simulink model "pfb_fir_real_test"  (Simulink 7.4)
settings: Solver=VariableStepDiscrete  StartTime=0.0  StopTime=500  RelTol=1e-3
libraries: xbsIndex_r4 x110
settings Model: Creator=User  LastModifiedBy=sgowda
settings OptimizationCC: InitFltsAndDblsToZero=on
settings DebuggingCC: SaveWithDisabledLinksMsg=none  SaveWithParameterizedLinksMsg=none

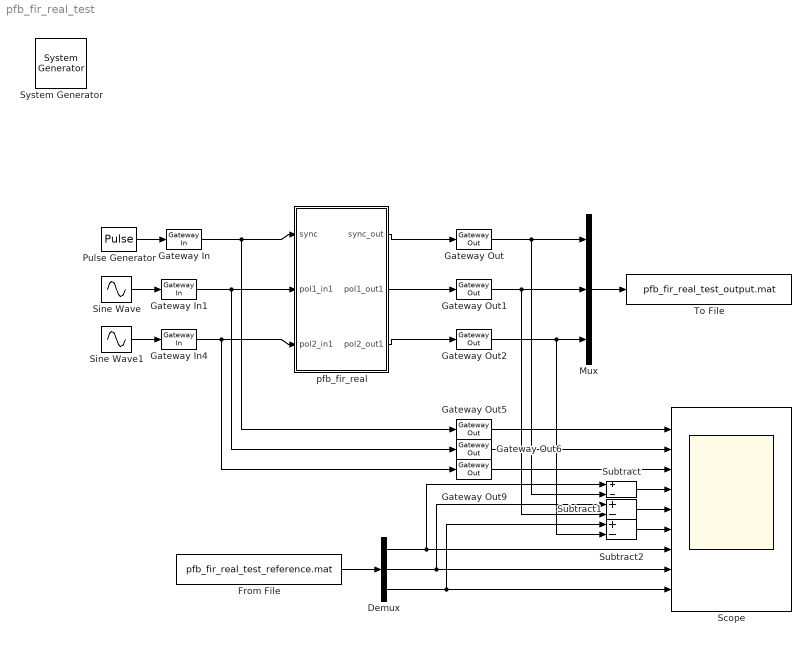
== system pfb_fir_real_test ==
  " System Generator" : xbsIndex_r4/ System Generator  Tag=genX  SystemSampleTime=-1  xilinxfamily=virtex4  part=xc4vsx35  speed=-10  package=ff668  synthesis_tool=XST  clock_wrapper=Clock Enables  directory=./netlist  testbench=off  simulink_period=1  sysclk_period=100  dcm_input_clock_period=100  incr_netlist=off  trim_vbits=Everywhere in SubSystem  dbl_ovrd=According to Block Masks  core_generation=According to Block Masks  run_coregen=off  deprecated_control=off  eval_field=0  block_type=sysgen
      settings: block_version=10.1.1
  Demux : Demux  Outputs=3
  From File : FromFile  FileName=pfb_fir_real_test_reference.mat  SampleTime=1
  Gateway In : xbsIndex_r4/Gateway In  arith_type=Boolean  n_bits=16  bin_pt=14  quantization="Round  (unbiased: +/- Inf)"  overflow=Saturate  period=1  dbl_ovrd=off  timing_constraint=None  locs_specified=off  LOCs={}  hdl_port=on  block_type=gatewayin
      settings: infoedit="Gateway in block.  Converts inputs of type Simulink integer, double and fixed point to  Xilinx fixed point type.<P><P>Hardware notes:  In hardware these blocks become top level input ports."  block_version=10.1.1
  Gateway In1 : xbsIndex_r4/Gateway In  arith_type="Signed  (2's comp)"  n_bits=10  bin_pt=9  quantization=Truncate  overflow=Wrap  period=1  dbl_ovrd=off  timing_constraint=None  locs_specified=off  LOCs={}  hdl_port=on  block_type=gatewayin
      settings: infoedit="Gateway in block.  Converts inputs of type Simulink integer, double and fixed point to  Xilinx fixed point type.<P><P>Hardware notes:  In hardware these blocks become top level input ports."  block_version=10.1.1
  Gateway In4 : xbsIndex_r4/Gateway In  arith_type="Signed  (2's comp)"  n_bits=10  bin_pt=9  quantization=Truncate  overflow=Wrap  period=1  dbl_ovrd=off  timing_constraint=None  locs_specified=off  LOCs={}  hdl_port=on  block_type=gatewayin
      settings: infoedit="Gateway in block.  Converts inputs of type Simulink integer, double and fixed point to  Xilinx fixed point type.<P><P>Hardware notes:  In hardware these blocks become top level input ports."  block_version=10.1.1
  Gateway Out{,1..2,5..6,9} (6 alike) : xbsIndex_r4/Gateway Out  hdl_port=on  timing_constraint=None  locs_specified=off  LOCs={}  block_type=gatewayout
      settings: infoedit="Gateway out block.  Converts Xilinx fixed point inputs into ouputs of type Simulink integer, double, or fixed point.<P><P>Hardware notes:  In hardware these blocks become top level output ports or are discarded, depending on how they are configured."  block_version=10.1.1
  Mux : Mux  Inputs=3
  Pulse Generator : DiscretePulseGenerator  Amplitude=1  Period=2^8  PulseWidth=1  PhaseDelay=13  SampleTime=1
  Scope : Scope  NumInputPorts=9
      settings: YMin=-5~-5~-5~-5~-5~-5~-5~-5~-5  YMax=5~5~5~5~5~5~5~5~5
  Sine Wave : Sin  SineType=Sample based  Amplitude=0.8  Bias=0  Frequency=1  Phase=0  Samples=16  SampleTime=1  Offset=7
  Sine Wave1 : Sin  SineType=Sample based  Amplitude=0.8  Bias=0  Frequency=1  Phase=0  Samples=8  SampleTime=1  Offset=7
  Subtract : Sum  Inputs=+-  OutDataType=fixdt(1, 16)  OutScaling=2^-10
  Subtract1 : Sum  Inputs=+-  OutDataType=fixdt(1, 16)  OutScaling=2^-10
  Subtract2 : Sum  Inputs=+-  OutDataType=fixdt(1, 16)  OutScaling=2^-10
  To File : ToFile  Filename=pfb_fir_real_test_output.mat  MatrixName=output
  pfb_fir_real : Subsystem  mask(pfb_fir_real){PFBSize=5, TotalTaps=5, WindowType=chebwin, n_inputs=0, MakeBiplex=1, BitWidthIn=10, BitWidthOut=22, CoeffBitWidth=10, CoeffDistMem=0, add_latency=2, mult_latency=3, bram_latency=1, conv_latency=2, quantization=Truncate, fwidth=0.80000000000000004440892098500626, specify_mult=off, mult_spec=[2                                      2], adder_folding=on, adder_tree_impl=Fabric}
      mask prompts: PFBSize "Size of PFB: (2^? pnts)"; TotalTaps "Total Number of Taps:"; WindowType "Windowing Function:"; n_inputs "Number of Simultaneous Inputs: (2^?)"; MakeBiplex "Make Biplex"; BitWidthIn "Input Bitwidth:"; BitWidthOut "Output Bitwidth:"; CoeffBitWidth "Coefficient Bitwidth:"; CoeffDistMem "Use Distributed Memory for Coeffs"; add_latency "Add Latency"; mult_latency "Mult Latency"; bram_latency "BRAM Latency"; conv_latency "Convert latency"; quantization "Quantization Behavior"; fwidth "Bin Width Scaling (normal=1)"; specify_mult "Specify multiplier use (behavioral if not specified)"; mult_spec "Multiplier specification (0=core, 1=embedded, 2=behavioural) (left=1st tap)"; adder_folding "Fold adders into DSPs"; adder_tree_impl "Adder implementation"
      mask help:
      | Fold adders into DSPs: Causes adders to be absorbed into DSP blocks (supported in Virtex5)
      | Adder implementation: Cores using Fabric or DSP48 or behavioral HDL
      mask init:
      | config.source = str2func('pfb_fir_init_xblock');
      | config.toplevel = gcb;
      | config.depend = {'pfb_fir_init_xblock.m', 'pfb_row_init_xblock.m', ...
      |     'adder_tree_init_xblock.m', 'macc_dsp48e_init_xblock.m', ...
      |     'pfb_coeff_gen_init_xblock.m', 'simd_add_dsp48e_init_xblock.m', ...
      |     'tap_multiply_fabric_init_xblock'};
      | if strcmp(specify_mult, 'on')
      |     mult_impl = 'DSP48e';
      | else
      |     mult_impl = 'Fabric';
      | end
      | xBlock(config, {PFBSize, TotalTaps, WindowType, ...
      |     n_inputs, MakeBiplex, BitWidthIn, BitWidthOut, ...
      |     CoeffBitWidth, CoeffDistMem, add_latency, mult_latency, ...
      |     bram_latency, conv_latency, quantization, fwidth, ...
      |     adder_tree_impl, mult_impl});
      settings: AttributesFormatString=taps=2, add_latency=1
      mask Help: eval('xlWeb(''http://casper.berkeley.edu/wiki/Pfb_fir_real'')')
      mask StyleString: edit,edit,popup(bartlett|barthannwin|blackman|blackmanharris|bohamwin|chebwin|flattopwin|gausswin|hamming|hann|kaiser|nuttallwin|parzenwin|rectwin|tukeywin|triang|userwindow),edit,edit,edit,edit,edit,edit,edit,edit,edit,edit,popup(Truncate|Round  (unbiased: +/- Inf)|Round  (unbiased: Even Values)),edit,checkbox,edit,checkbox,popup(Behavioral|Fabric|DSP48e)
      mask CallbackString:
      | |%num_taps = eval(get_param(gcb, 'TotalTaps'));
      | %old_vec = eval(get_param(gcb, 'mult_spec'));=-0l
      | 
      | %vec = 2.*ones(1,num_taps);
      | %old_size = length(old_vec);
      | 
      | %if(old_size <= num_taps),
      | %    new_size = old_size;
      | %else,
      | %    new_size = num_taps;
      | %end
      | 
      | %for n = 1:new_size, vec(n) = old_vec(n); end
      | %set_param(gcb, 'mult_spec', mat2str(vec));||||||||||||||%thisVariable = 'specify_mult';
      | %affectedVars = {'mult_spec'};
      | 
      | %thisBlock = gcb();
      | %thisVarState = get_param(thisBlock, thisVariable);
      | %maskNames = get_param(thisBlock, 'MaskNames');
      | %maskEnables = get_param(thisBlock, 'MaskEnables');
      | 
      | %for varName = affectedVars
      | %    varIndex = find(ismember(maskNames, varName));
      | %    maskEnables{varIndex} = thisVarState;
      | %end
      | 
      | %set_param(thisBlock, 'MaskEnables', maskEnables);|||
  wires:
  Pulse Generator/1 -> Gateway In/1
  Gateway In/1 -> Gateway Out5/1, pfb_fir_real/1(sync)
  Sine Wave/1 -> Gateway In1/1
  pfb_fir_real/1(sync_out) -> Gateway Out/1
  Sine Wave1/1 -> Gateway In4/1
  Gateway In1/1 -> Gateway Out6/1, pfb_fir_real/2(pol1_in1)
  Gateway In4/1 -> Gateway Out9/1, pfb_fir_real/3(pol2_in1)
  Gateway Out5/1 -> Scope/1
  Gateway Out6/1 -> Scope/2
  Gateway Out/1 -> Mux/1, Subtract/2
  Gateway Out1/1 -> Mux/2, Subtract1/2
  Gateway Out2/1 -> Mux/3, Subtract2/2
  Mux/1 -> To File/1
  pfb_fir_real/3(pol2_out1) -> Gateway Out2/1
  pfb_fir_real/2(pol1_out1) -> Gateway Out1/1
  Gateway Out9/1 -> Scope/3
  Subtract/1 -> Scope/4
  Subtract1/1 -> Scope/5
  Subtract2/1 -> Scope/6
  From File/1 -> Demux/1
  Demux/1 -> Scope/7, Subtract/1
  Demux/2 -> Scope/8, Subtract1/1
  Demux/3 -> Scope/9, Subtract2/1

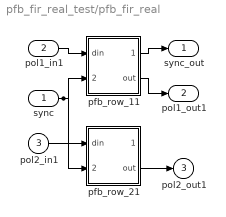
== system pfb_fir_real_test/pfb_fir_real ==
  sync : Inport
  pol1_in1 : Inport  Port=2
  pol2_in1 : Inport  Port=3
  pfb_row_11 : Subsystem
  pfb_row_21 : Subsystem
  sync_out : Outport
  pol1_out1 : Outport  Port=2
  pol2_out1 : Outport  Port=3
  wires:
  sync/1 -> pfb_row_21/2(sync), pfb_row_11/2(sync)
  pfb_row_21/2(out) -> pol2_out1/1
  pol2_in1/1 -> pfb_row_21/1(din)
  pfb_row_11/2(out) -> pol1_out1/1
  pfb_row_11/1(sync_out) -> sync_out/1
  pol1_in1/1 -> pfb_row_11/1(din)

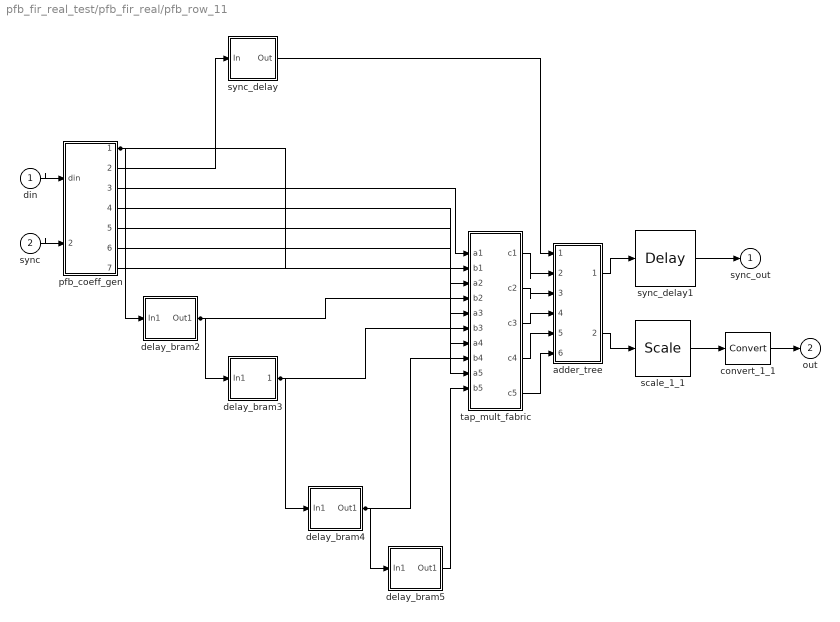
== system pfb_fir_real_test/pfb_fir_real/pfb_row_11 ==
  din : Inport
  sync : Inport  Port=2
  adder_tree : Subsystem
  convert_1_1 : xbsIndex_r4/Convert  arith_type="Signed  (2's comp)"  n_bits=22  bin_pt=21  quantization="Round  (unbiased: +/- Inf)"  overflow=Saturate  latency=1  dbl_ovrd=off  pipeline=on  block_type=convert
      settings: block_version=11.4
  delay_bram2 : Subsystem
  delay_bram3 : Subsystem
  delay_bram4 : Subsystem
  delay_bram5 : Subsystem
  pfb_coeff_gen : Subsystem
  scale_1_1 : xbsIndex_r4/Scale  scale_factor=-4  dbl_ovrd=off  block_type=scale
  sync_delay : Subsystem
  sync_delay1 : xbsIndex_r4/Delay  en=off  latency=2  dbl_ovrd=off  reg_retiming=off  block_type=delay
      settings: block_version=11.4
  tap_mult_fabric : Subsystem
  sync_out : Outport
  out : Outport  Port=2
  wires:
  pfb_coeff_gen/1(dout) -> tap_mult_fabric/2(b1), delay_bram2/1(In1)
  delay_bram2/1(Out1) -> tap_mult_fabric/4(b2), delay_bram3/1(In1)
  delay_bram3/1(Out1) -> tap_mult_fabric/6(b3), delay_bram4/1(In1)
  delay_bram4/1(Out1) -> tap_mult_fabric/8(b4), delay_bram5/1(In1)
  sync_delay/1(Out) -> adder_tree/1(sync)
  pfb_coeff_gen/2(sync_out) -> sync_delay/1(In)
  adder_tree/2(dout) -> scale_1_1/1
  adder_tree/1(sync_out) -> sync_delay1/1
  tap_mult_fabric/5(c5) -> adder_tree/6(din_5)
  tap_mult_fabric/4(c4) -> adder_tree/5(din_4)
  tap_mult_fabric/3(c3) -> adder_tree/4(din_3)
  tap_mult_fabric/2(c2) -> adder_tree/3(din_2)
  tap_mult_fabric/1(c1) -> adder_tree/2(din_1)
  delay_bram5/1(Out1) -> tap_mult_fabric/10(b5)
  pfb_coeff_gen/7(coeffs5) -> tap_mult_fabric/9(a5)
  pfb_coeff_gen/6(coeffs4) -> tap_mult_fabric/7(a4)
  pfb_coeff_gen/5(coeffs3) -> tap_mult_fabric/5(a3)
  pfb_coeff_gen/4(coeffs2) -> tap_mult_fabric/3(a2)
  pfb_coeff_gen/3(coeffs1) -> tap_mult_fabric/1(a1)
  sync_delay1/1 -> sync_out/1
  scale_1_1/1 -> convert_1_1/1
  convert_1_1/1 -> out/1
  sync/1 -> pfb_coeff_gen/2(sync)
  din/1 -> pfb_coeff_gen/1(din)

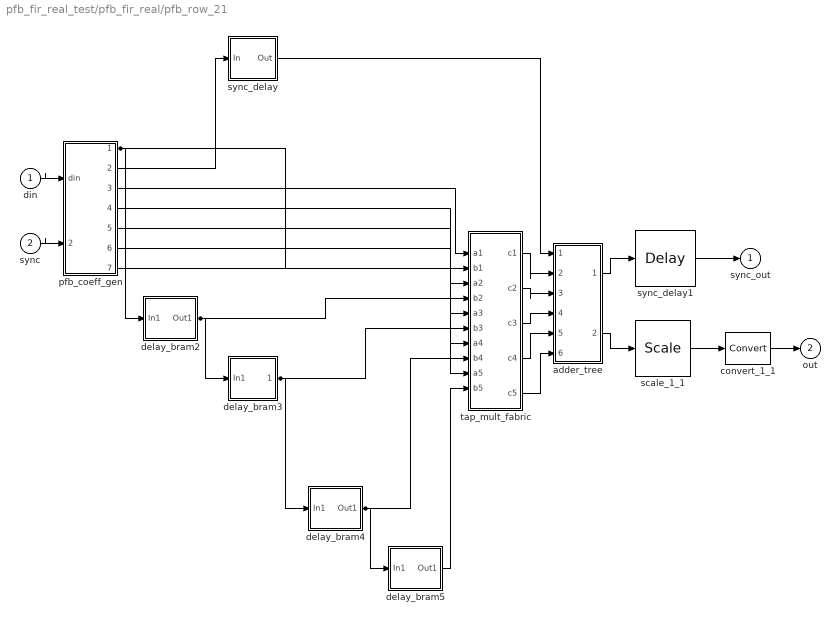
== system pfb_fir_real_test/pfb_fir_real/pfb_row_21 ==
  din : Inport
  sync : Inport  Port=2
  adder_tree : Subsystem
  convert_1_1 : xbsIndex_r4/Convert  arith_type="Signed  (2's comp)"  n_bits=22  bin_pt=21  quantization="Round  (unbiased: +/- Inf)"  overflow=Saturate  latency=1  dbl_ovrd=off  pipeline=on  block_type=convert
      settings: block_version=11.4
  delay_bram2 : Subsystem
  delay_bram3 : Subsystem
  delay_bram4 : Subsystem
  delay_bram5 : Subsystem
  pfb_coeff_gen : Subsystem
  scale_1_1 : xbsIndex_r4/Scale  scale_factor=-4  dbl_ovrd=off  block_type=scale
  sync_delay : Subsystem
  sync_delay1 : xbsIndex_r4/Delay  en=off  latency=2  dbl_ovrd=off  reg_retiming=off  block_type=delay
      settings: block_version=11.4
  tap_mult_fabric : Subsystem
  sync_out : Outport
  out : Outport  Port=2
  wires:
  pfb_coeff_gen/1(dout) -> tap_mult_fabric/2(b1), delay_bram2/1(In1)
  delay_bram2/1(Out1) -> tap_mult_fabric/4(b2), delay_bram3/1(In1)
  delay_bram3/1(Out1) -> tap_mult_fabric/6(b3), delay_bram4/1(In1)
  delay_bram4/1(Out1) -> tap_mult_fabric/8(b4), delay_bram5/1(In1)
  sync_delay/1(Out) -> adder_tree/1(sync)
  pfb_coeff_gen/2(sync_out) -> sync_delay/1(In)
  adder_tree/2(dout) -> scale_1_1/1
  adder_tree/1(sync_out) -> sync_delay1/1
  tap_mult_fabric/5(c5) -> adder_tree/6(din_5)
  tap_mult_fabric/4(c4) -> adder_tree/5(din_4)
  tap_mult_fabric/3(c3) -> adder_tree/4(din_3)
  tap_mult_fabric/2(c2) -> adder_tree/3(din_2)
  tap_mult_fabric/1(c1) -> adder_tree/2(din_1)
  delay_bram5/1(Out1) -> tap_mult_fabric/10(b5)
  pfb_coeff_gen/7(coeffs5) -> tap_mult_fabric/9(a5)
  pfb_coeff_gen/6(coeffs4) -> tap_mult_fabric/7(a4)
  pfb_coeff_gen/5(coeffs3) -> tap_mult_fabric/5(a3)
  pfb_coeff_gen/4(coeffs2) -> tap_mult_fabric/3(a2)
  pfb_coeff_gen/3(coeffs1) -> tap_mult_fabric/1(a1)
  sync_delay1/1 -> sync_out/1
  scale_1_1/1 -> convert_1_1/1
  convert_1_1/1 -> out/1
  sync/1 -> pfb_coeff_gen/2(sync)
  din/1 -> pfb_coeff_gen/1(din)

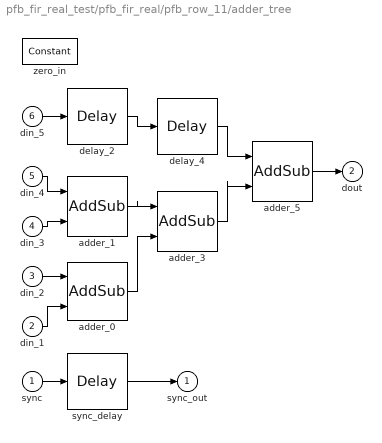
== system pfb_fir_real_test/pfb_fir_real/pfb_row_11/adder_tree ==
  sync : Inport
  din_1 : Inport  Port=2
  din_2 : Inport  Port=3
  din_3 : Inport  Port=4
  din_4 : Inport  Port=5
  din_5 : Inport  Port=6
  adder_{0..1,3,5} (4 alike) : xbsIndex_r4/AddSub  mode=Addition  use_carryin=off  use_carryout=off  en=off  latency=2  precision=Full  arith_type=Unsigned  n_bits=16  bin_pt=14  quantization=Truncate  overflow=Wrap  dbl_ovrd=off  use_behavioral_HDL=off  hw_selection=Fabric  pipelined=off  block_type=addsub
  delay_2 : xbsIndex_r4/Delay  en=off  latency=2  dbl_ovrd=off  reg_retiming=off  block_type=delay
      settings: block_version=11.4
  delay_4 : xbsIndex_r4/Delay  en=off  latency=2  dbl_ovrd=off  reg_retiming=off  block_type=delay
      settings: block_version=11.4
  sync_delay : xbsIndex_r4/Delay  en=off  latency=6  dbl_ovrd=off  reg_retiming=off  block_type=delay
      settings: block_version=11.4
  zero_in : xbsIndex_r4/Constant  arith_type=Unsigned  const=0  n_bits=18  bin_pt=17  explicit_period=off  period=1  equ=P=C  opselect=C  inp2=PCIN>>17  opr=+  inp1=P  carry=CIN  dbl_ovrd=off  block_type=constant
      settings: block_version=11.4
  sync_out : Outport
  dout : Outport  Port=2
  wires:
  adder_5/1 -> dout/1
  adder_3/1 -> adder_5/2
  delay_4/1 -> adder_5/1
  delay_2/1 -> delay_4/1
  adder_0/1 -> adder_3/2
  adder_1/1 -> adder_3/1
  din_5/1 -> delay_2/1
  din_3/1 -> adder_1/2
  din_4/1 -> adder_1/1
  din_1/1 -> adder_0/2
  din_2/1 -> adder_0/1
  sync_delay/1 -> sync_out/1
  sync/1 -> sync_delay/1

== system pfb_fir_real_test/pfb_fir_real/pfb_row_11/delay_bram2 ==
  In1 : Inport
  Constant2 : xbsIndex_r4/Constant  arith_type=Boolean  const=1  n_bits=1  bin_pt=0  explicit_period=on  period=1  equ=P=C  opselect=C  inp2=PCIN>>17  opr=+  inp1=P  carry=CIN  dbl_ovrd=off  block_type=constant
      settings: block_version=11.4
  Counter : xbsIndex_r4/Counter  cnt_type=Count Limited  cnt_to=30  operation=Up  start_count=0  cnt_by_val=1  arith_type=Unsigned  n_bits=5  bin_pt=0  load_pin=off  rst=off  en=off  explicit_period=on  period=1  dbl_ovrd=off  use_behavioral_HDL=off  implementation=DSP48  use_rpm=on  block_type=counter
      settings: block_version=11.4
  Single Port RAM : xbsIndex_r4/Single Port RAM  depth=32  initVector=0  distributed_mem=Block RAM  write_mode=Read Before Write  rst=off  init_reg=0  en=off  latency=1  dbl_ovrd=off  optimize=Area  use_rpm=off  block_type=spram
  Out1 : Outport
  wires:
  Single Port RAM/1 -> Out1/1
  Constant2/1 -> Single Port RAM/3
  In1/1 -> Single Port RAM/2
  Counter/1 -> Single Port RAM/1

== system pfb_fir_real_test/pfb_fir_real/pfb_row_11/delay_bram3 ==
  In1 : Inport
  Constant2 : xbsIndex_r4/Constant  arith_type=Boolean  const=1  n_bits=1  bin_pt=0  explicit_period=on  period=1  equ=P=C  opselect=C  inp2=PCIN>>17  opr=+  inp1=P  carry=CIN  dbl_ovrd=off  block_type=constant
      settings: block_version=11.4
  Counter : xbsIndex_r4/Counter  cnt_type=Count Limited  cnt_to=30  operation=Up  start_count=0  cnt_by_val=1  arith_type=Unsigned  n_bits=5  bin_pt=0  load_pin=off  rst=off  en=off  explicit_period=on  period=1  dbl_ovrd=off  use_behavioral_HDL=off  implementation=DSP48  use_rpm=on  block_type=counter
      settings: block_version=11.4
  Single Port RAM : xbsIndex_r4/Single Port RAM  depth=32  initVector=0  distributed_mem=Block RAM  write_mode=Read Before Write  rst=off  init_reg=0  en=off  latency=1  dbl_ovrd=off  optimize=Area  use_rpm=off  block_type=spram
  Out1 : Outport
  wires:
  Single Port RAM/1 -> Out1/1
  Constant2/1 -> Single Port RAM/3
  In1/1 -> Single Port RAM/2
  Counter/1 -> Single Port RAM/1

== system pfb_fir_real_test/pfb_fir_real/pfb_row_11/delay_bram4 ==
  In1 : Inport
  Constant2 : xbsIndex_r4/Constant  arith_type=Boolean  const=1  n_bits=1  bin_pt=0  explicit_period=on  period=1  equ=P=C  opselect=C  inp2=PCIN>>17  opr=+  inp1=P  carry=CIN  dbl_ovrd=off  block_type=constant
      settings: block_version=11.4
  Counter : xbsIndex_r4/Counter  cnt_type=Count Limited  cnt_to=30  operation=Up  start_count=0  cnt_by_val=1  arith_type=Unsigned  n_bits=5  bin_pt=0  load_pin=off  rst=off  en=off  explicit_period=on  period=1  dbl_ovrd=off  use_behavioral_HDL=off  implementation=DSP48  use_rpm=on  block_type=counter
      settings: block_version=11.4
  Single Port RAM : xbsIndex_r4/Single Port RAM  depth=32  initVector=0  distributed_mem=Block RAM  write_mode=Read Before Write  rst=off  init_reg=0  en=off  latency=1  dbl_ovrd=off  optimize=Area  use_rpm=off  block_type=spram
  Out1 : Outport
  wires:
  Single Port RAM/1 -> Out1/1
  Constant2/1 -> Single Port RAM/3
  In1/1 -> Single Port RAM/2
  Counter/1 -> Single Port RAM/1

== system pfb_fir_real_test/pfb_fir_real/pfb_row_11/delay_bram5 ==
  In1 : Inport
  Constant2 : xbsIndex_r4/Constant  arith_type=Boolean  const=1  n_bits=1  bin_pt=0  explicit_period=on  period=1  equ=P=C  opselect=C  inp2=PCIN>>17  opr=+  inp1=P  carry=CIN  dbl_ovrd=off  block_type=constant
      settings: block_version=11.4
  Counter : xbsIndex_r4/Counter  cnt_type=Count Limited  cnt_to=30  operation=Up  start_count=0  cnt_by_val=1  arith_type=Unsigned  n_bits=5  bin_pt=0  load_pin=off  rst=off  en=off  explicit_period=on  period=1  dbl_ovrd=off  use_behavioral_HDL=off  implementation=DSP48  use_rpm=on  block_type=counter
      settings: block_version=11.4
  Single Port RAM : xbsIndex_r4/Single Port RAM  depth=32  initVector=0  distributed_mem=Block RAM  write_mode=Read Before Write  rst=off  init_reg=0  en=off  latency=1  dbl_ovrd=off  optimize=Area  use_rpm=off  block_type=spram
  Out1 : Outport
  wires:
  Single Port RAM/1 -> Out1/1
  Constant2/1 -> Single Port RAM/3
  In1/1 -> Single Port RAM/2
  Counter/1 -> Single Port RAM/1

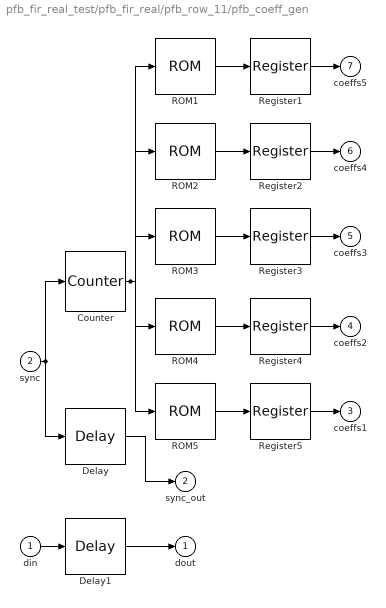
== system pfb_fir_real_test/pfb_fir_real/pfb_row_11/pfb_coeff_gen ==
  din : Inport
  sync : Inport  Port=2
  Counter : xbsIndex_r4/Counter  cnt_type=Free Running  cnt_to=Inf  operation=Up  start_count=0  cnt_by_val=1  arith_type=Unsigned  n_bits=5  bin_pt=0  load_pin=off  rst=on  en=off  explicit_period=on  period=1  dbl_ovrd=off  use_behavioral_HDL=off  implementation=Fabric  use_rpm=on  block_type=counter
      settings: block_version=11.4
  Delay : xbsIndex_r4/Delay  en=off  latency=2  dbl_ovrd=off  reg_retiming=off  block_type=delay
      settings: block_version=11.4
  Delay1 : xbsIndex_r4/Delay  en=off  latency=3  dbl_ovrd=off  reg_retiming=off  block_type=delay
      settings: block_version=11.4
  ROM1 : xbsIndex_r4/ROM  depth=32  initVector=[-1.83537948689192e-20 -5.5570212494937e-06 -1.63600419269467e-05 -3.47242296265235e-05 -6.35238166447315e-05 -0.000106241976471681 -0.000167008217876277 -0.000250618800937326 -0.000362535388329735 -0.000508856971932249 -0.000696260082747423 -0.000931902422689507 -0.00122328536860849 -0.00157807130674446 -0.00200385246963349 -0.002507868871658 -0.00309667407189773 -0.00377574882462827 -0.00454906419223727 -0.00541859736832988 -0.00638380525859058 -0.00744106275440964 -0.00858307456340268 -0.00979827137977639 -0.011070203029117 -0.0123769429460894 -0.0136905198771712 -0.0149763939810333 -0.0161929954652235 -0.017291344491685 -0.0182147712532231 -0.0188987548237974]  distributed_mem=Block RAM  rst=off  init_reg=0  en=off  latency=2  arith_type="Signed  (2's comp)"  n_bits=10  bin_pt=9  dbl_ovrd=off  optimize=Area  use_rpm=on  block_type=sprom
      settings: block_version=11.4
  ROM2 : xbsIndex_r4/ROM  depth=32  initVector=[-0.0192708985824556 -0.0192510586801436 -0.0187516401496287 -0.0176780728545899 -0.0159294765527955 -0.013399520943983 -0.00997748273503472 -0.00554949754803241 9.58776090258162e-18 0.00678665941101795 0.0149244367666534 0.024523677457147 0.0356890847292955 0.0485176039711326 0.0630962566317489 0.0794999611480237 0.0977893811012691 0.118008842950763 0.140184366995717 0.164321855626379 0.190405482381545 0.21839632379788 0.248231273503403 0.279822274484999 0.313055900984824 0.34779331611502 0.383870625110952 0.421099637279897 0.459269042275782 0.498145998490477 0.537478123262804 0.576995866443847]  distributed_mem=Block RAM  rst=off  init_reg=0  en=off  latency=2  arith_type="Signed  (2's comp)"  n_bits=10  bin_pt=9  dbl_ovrd=off  optimize=Area  use_rpm=on  block_type=sprom
      settings: block_version=11.4
  ROM3 : xbsIndex_r4/ROM  depth=32  initVector=[0.616415240804449 0.655440875013837 0.693769347641133 0.731092754011235 0.767102451949175 0.80149292762253 0.83396571896988 0.864233331691149 0.892023081552472 0.917080796874454 0.939174316547831 0.958096721742031 0.973669243595624 0.98574379452744 0.99420507727783 0.998972233248538 1 0.997279356709406 0.990837645797992 0.980738168597035 0.967079262627824 0.949992877609162 0.929642676468857 0.906221696224427 0.879949611428438 0.851069649779872 0.819845215341666 0.786556279459168 0.751495602856677 0.714964854442019 0.67727069304653 0.638720877676221]  distributed_mem=Block RAM  rst=off  init_reg=0  en=off  latency=2  arith_type="Signed  (2's comp)"  n_bits=10  bin_pt=9  dbl_ovrd=off  optimize=Area  use_rpm=on  block_type=sprom
      settings: block_version=11.4
  ROM4 : xbsIndex_r4/ROM  depth=32  initVector=[0.599620469886999 0.560268188690169 0.520952974039709 0.481950809570252 0.443521848986383 0.40590788350912 0.369330180237019 0.333987713358341 0.300055802042386 0.267685160726547 0.237001359579851 0.208104685332775 0.181070385572542 0.155949273151139 0.132768661658431 0.111533598070868 0.0922283547694533 0.0748181401760309 0.0592509853065098 0.0454597625806334 0.0333642932339546 0.0228735006003976 0.0138875683049731 0.00630006494050392 8.87861210313256e-18 -0.00512622041298097 -0.00919296538822508 -0.0123137013214723 -0.0145994824432491 -0.0161576231160187 -0.0170905605431562 -0.017494911978617]  distributed_mem=Block RAM  rst=off  init_reg=0  en=off  latency=2  arith_type="Signed  (2's comp)"  n_bits=10  bin_pt=9  dbl_ovrd=off  optimize=Area  use_rpm=on  block_type=sprom
      settings: block_version=11.4
  ROM5 : xbsIndex_r4/ROM  depth=32  initVector=[-0.017460726222102 -0.0170709252152087 -0.0164009279898009 -0.0155184461159748 -0.0144834371934731 -0.013348200851566 -0.0121576001774965 -0.0109493904773777 -0.00975463676747319 -0.00859820136776993 -0.00749928338318453 -0.00647199266182947 -0.00552594195933946 -0.00466684245382657 -0.00389708938574173 -0.00321632637849668 -0.00262197886823068 -0.00210974897665909 -0.00167406604597449 -0.00130848887129482 -0.00100605737264354 -0.000759593010482301 -0.000561948639457462 -0.000406209694920779 -0.000285849604064716 -0.000194843103417715 -0.000127741728803638 -7.97161304010817e-05 -4.65700670323589e-05 -2.47309672256418e-05 -1.12218300973319e-05 -5.95375857785367e-06]  distributed_mem=Block RAM  rst=off  init_reg=0  en=off  latency=2  arith_type="Signed  (2's comp)"  n_bits=10  bin_pt=9  dbl_ovrd=off  optimize=Area  use_rpm=on  block_type=sprom
      settings: block_version=11.4
  Register{1..5} (5 alike) : xbsIndex_r4/Register  init=0  rst=off  en=off  dbl_ovrd=off  block_type=register
      settings: block_version=11.4
  dout : Outport
  sync_out : Outport  Port=2
  coeffs1 : Outport  Port=3
  coeffs2 : Outport  Port=4
  coeffs3 : Outport  Port=5
  coeffs4 : Outport  Port=6
  coeffs5 : Outport  Port=7
  wires:
  sync/1 -> Delay/1, Counter/1
  Counter/1 -> ROM1/1, ROM2/1, ROM3/1, ROM4/1, ROM5/1
  Register1/1 -> coeffs5/1
  ROM1/1 -> Register1/1
  Register2/1 -> coeffs4/1
  ROM2/1 -> Register2/1
  Register3/1 -> coeffs3/1
  ROM3/1 -> Register3/1
  Register4/1 -> coeffs2/1
  ROM4/1 -> Register4/1
  Register5/1 -> coeffs1/1
  ROM5/1 -> Register5/1
  Delay1/1 -> dout/1
  din/1 -> Delay1/1
  Delay/1 -> sync_out/1

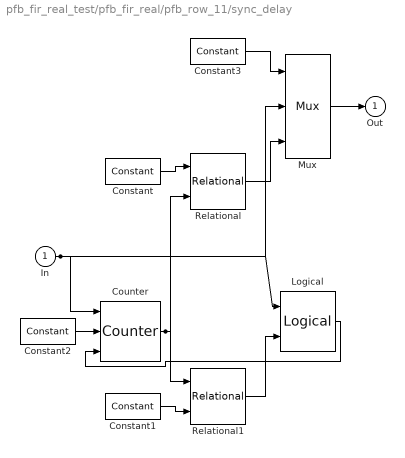
== system pfb_fir_real_test/pfb_fir_real/pfb_row_11/sync_delay ==
  In : Inport
  Constant : xbsIndex_r4/Constant  arith_type=Unsigned  const=1  n_bits=8  bin_pt=0  explicit_period=on  period=1  equ=P=C  opselect=C  inp2=PCIN>>17  opr=+  inp1=P  carry=CIN  dbl_ovrd=off  block_type=constant
      settings: block_version=11.4
  Constant1 : xbsIndex_r4/Constant  arith_type=Unsigned  const=0  n_bits=8  bin_pt=0  explicit_period=on  period=1  equ=P=C  opselect=C  inp2=PCIN>>17  opr=+  inp1=P  carry=CIN  dbl_ovrd=off  block_type=constant
      settings: block_version=11.4
  Constant2 : xbsIndex_r4/Constant  arith_type=Unsigned  const=131  n_bits=8  bin_pt=0  explicit_period=on  period=1  equ=P=C  opselect=C  inp2=PCIN>>17  opr=+  inp1=P  carry=CIN  dbl_ovrd=off  block_type=constant
      settings: block_version=11.4
  Constant3 : xbsIndex_r4/Constant  arith_type=Unsigned  const=1  n_bits=1  bin_pt=0  explicit_period=on  period=1  equ=P=C  opselect=C  inp2=PCIN>>17  opr=+  inp1=P  carry=CIN  dbl_ovrd=off  block_type=constant
      settings: block_version=11.4
  Counter : xbsIndex_r4/Counter  cnt_type=Free Running  cnt_to=Inf  operation=Down  start_count=0  cnt_by_val=1  arith_type=Unsigned  n_bits=8  bin_pt=0  load_pin=on  rst=off  en=on  explicit_period=on  period=1  dbl_ovrd=off  use_behavioral_HDL=off  implementation=Fabric  use_rpm=on  block_type=counter
      settings: block_version=11.4
  Logical : xbsIndex_r4/Logical  logical_function=OR  inputs=2  en=off  latency=0  precision=Full  arith_type=Unsigned  n_bits=16  bin_pt=0  align_bp=on  dbl_ovrd=off  block_type=logical
      settings: block_version=11.4
  Mux : xbsIndex_r4/Mux  inputs=2  en=off  latency=0  precision=Full  arith_type="Signed  (2's comp)"  n_bits=8  bin_pt=2  quantization=Truncate  overflow=Wrap  dbl_ovrd=off  block_type=mux
      settings: block_version=11.4
  Relational : xbsIndex_r4/Relational  mode=a=b  en=off  latency=0  dbl_ovrd=off  block_type=relational
  Relational1 : xbsIndex_r4/Relational  mode=a!=b  en=off  latency=0  dbl_ovrd=off  block_type=relational
  Out : Outport
  wires:
  In/1 -> Mux/2, Logical/1, Counter/1
  Counter/1 -> Relational1/1, Relational/2
  Relational1/1 -> Logical/2
  Constant1/1 -> Relational1/2
  Relational/1 -> Mux/3
  Constant/1 -> Relational/1
  Mux/1 -> Out/1
  Constant3/1 -> Mux/1
  Logical/1 -> Counter/3
  Constant2/1 -> Counter/2

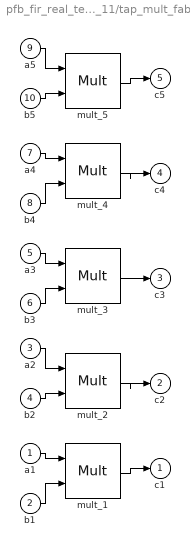
== system pfb_fir_real_test/pfb_fir_real/pfb_row_11/tap_mult_fabric ==
  a1 : Inport
  b1 : Inport  Port=2
  a2 : Inport  Port=3
  b2 : Inport  Port=4
  a3 : Inport  Port=5
  b3 : Inport  Port=6
  a4 : Inport  Port=7
  b4 : Inport  Port=8
  a5 : Inport  Port=9
  b5 : Inport  Port=10
  mult_{1..5} (5 alike) : xbsIndex_r4/Mult  precision=Full  arith_type="Signed  (2's comp)"  n_bits=16  bin_pt=14  quantization=Truncate  overflow=Wrap  en=off  latency=3  dbl_ovrd=off  use_behavioral_HDL=off  opt=Speed  use_embedded=on  optimum_pipeline=off  pipeline=on  use_rpm=on  placement_style=Triangular  block_type=mult
      settings: block_version=11.4
  c1 : Outport
  c2 : Outport  Port=2
  c3 : Outport  Port=3
  c4 : Outport  Port=4
  c5 : Outport  Port=5
  wires:
  mult_5/1 -> c5/1
  b5/1 -> mult_5/2
  a5/1 -> mult_5/1
  mult_4/1 -> c4/1
  b4/1 -> mult_4/2
  a4/1 -> mult_4/1
  mult_3/1 -> c3/1
  b3/1 -> mult_3/2
  a3/1 -> mult_3/1
  mult_2/1 -> c2/1
  b2/1 -> mult_2/2
  a2/1 -> mult_2/1
  mult_1/1 -> c1/1
  b1/1 -> mult_1/2
  a1/1 -> mult_1/1

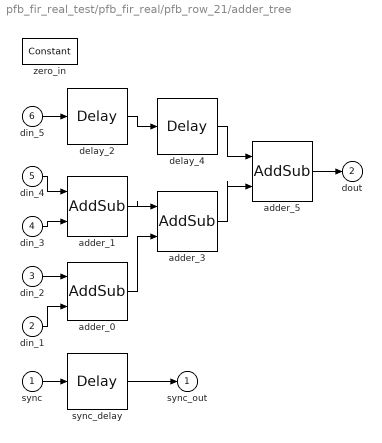
== system pfb_fir_real_test/pfb_fir_real/pfb_row_21/adder_tree ==
  sync : Inport
  din_1 : Inport  Port=2
  din_2 : Inport  Port=3
  din_3 : Inport  Port=4
  din_4 : Inport  Port=5
  din_5 : Inport  Port=6
  adder_{0..1,3,5} (4 alike) : xbsIndex_r4/AddSub  mode=Addition  use_carryin=off  use_carryout=off  en=off  latency=2  precision=Full  arith_type=Unsigned  n_bits=16  bin_pt=14  quantization=Truncate  overflow=Wrap  dbl_ovrd=off  use_behavioral_HDL=off  hw_selection=Fabric  pipelined=off  block_type=addsub
  delay_2 : xbsIndex_r4/Delay  en=off  latency=2  dbl_ovrd=off  reg_retiming=off  block_type=delay
      settings: block_version=11.4
  delay_4 : xbsIndex_r4/Delay  en=off  latency=2  dbl_ovrd=off  reg_retiming=off  block_type=delay
      settings: block_version=11.4
  sync_delay : xbsIndex_r4/Delay  en=off  latency=6  dbl_ovrd=off  reg_retiming=off  block_type=delay
      settings: block_version=11.4
  zero_in : xbsIndex_r4/Constant  arith_type=Unsigned  const=0  n_bits=18  bin_pt=17  explicit_period=off  period=1  equ=P=C  opselect=C  inp2=PCIN>>17  opr=+  inp1=P  carry=CIN  dbl_ovrd=off  block_type=constant
      settings: block_version=11.4
  sync_out : Outport
  dout : Outport  Port=2
  wires:
  adder_5/1 -> dout/1
  adder_3/1 -> adder_5/2
  delay_4/1 -> adder_5/1
  delay_2/1 -> delay_4/1
  adder_0/1 -> adder_3/2
  adder_1/1 -> adder_3/1
  din_5/1 -> delay_2/1
  din_3/1 -> adder_1/2
  din_4/1 -> adder_1/1
  din_1/1 -> adder_0/2
  din_2/1 -> adder_0/1
  sync_delay/1 -> sync_out/1
  sync/1 -> sync_delay/1

== system pfb_fir_real_test/pfb_fir_real/pfb_row_21/delay_bram2 ==
  In1 : Inport
  Constant2 : xbsIndex_r4/Constant  arith_type=Boolean  const=1  n_bits=1  bin_pt=0  explicit_period=on  period=1  equ=P=C  opselect=C  inp2=PCIN>>17  opr=+  inp1=P  carry=CIN  dbl_ovrd=off  block_type=constant
      settings: block_version=11.4
  Counter : xbsIndex_r4/Counter  cnt_type=Count Limited  cnt_to=30  operation=Up  start_count=0  cnt_by_val=1  arith_type=Unsigned  n_bits=5  bin_pt=0  load_pin=off  rst=off  en=off  explicit_period=on  period=1  dbl_ovrd=off  use_behavioral_HDL=off  implementation=DSP48  use_rpm=on  block_type=counter
      settings: block_version=11.4
  Single Port RAM : xbsIndex_r4/Single Port RAM  depth=32  initVector=0  distributed_mem=Block RAM  write_mode=Read Before Write  rst=off  init_reg=0  en=off  latency=1  dbl_ovrd=off  optimize=Area  use_rpm=off  block_type=spram
  Out1 : Outport
  wires:
  Single Port RAM/1 -> Out1/1
  Constant2/1 -> Single Port RAM/3
  In1/1 -> Single Port RAM/2
  Counter/1 -> Single Port RAM/1

== system pfb_fir_real_test/pfb_fir_real/pfb_row_21/delay_bram3 ==
  In1 : Inport
  Constant2 : xbsIndex_r4/Constant  arith_type=Boolean  const=1  n_bits=1  bin_pt=0  explicit_period=on  period=1  equ=P=C  opselect=C  inp2=PCIN>>17  opr=+  inp1=P  carry=CIN  dbl_ovrd=off  block_type=constant
      settings: block_version=11.4
  Counter : xbsIndex_r4/Counter  cnt_type=Count Limited  cnt_to=30  operation=Up  start_count=0  cnt_by_val=1  arith_type=Unsigned  n_bits=5  bin_pt=0  load_pin=off  rst=off  en=off  explicit_period=on  period=1  dbl_ovrd=off  use_behavioral_HDL=off  implementation=DSP48  use_rpm=on  block_type=counter
      settings: block_version=11.4
  Single Port RAM : xbsIndex_r4/Single Port RAM  depth=32  initVector=0  distributed_mem=Block RAM  write_mode=Read Before Write  rst=off  init_reg=0  en=off  latency=1  dbl_ovrd=off  optimize=Area  use_rpm=off  block_type=spram
  Out1 : Outport
  wires:
  Single Port RAM/1 -> Out1/1
  Constant2/1 -> Single Port RAM/3
  In1/1 -> Single Port RAM/2
  Counter/1 -> Single Port RAM/1

== system pfb_fir_real_test/pfb_fir_real/pfb_row_21/delay_bram4 ==
  In1 : Inport
  Constant2 : xbsIndex_r4/Constant  arith_type=Boolean  const=1  n_bits=1  bin_pt=0  explicit_period=on  period=1  equ=P=C  opselect=C  inp2=PCIN>>17  opr=+  inp1=P  carry=CIN  dbl_ovrd=off  block_type=constant
      settings: block_version=11.4
  Counter : xbsIndex_r4/Counter  cnt_type=Count Limited  cnt_to=30  operation=Up  start_count=0  cnt_by_val=1  arith_type=Unsigned  n_bits=5  bin_pt=0  load_pin=off  rst=off  en=off  explicit_period=on  period=1  dbl_ovrd=off  use_behavioral_HDL=off  implementation=DSP48  use_rpm=on  block_type=counter
      settings: block_version=11.4
  Single Port RAM : xbsIndex_r4/Single Port RAM  depth=32  initVector=0  distributed_mem=Block RAM  write_mode=Read Before Write  rst=off  init_reg=0  en=off  latency=1  dbl_ovrd=off  optimize=Area  use_rpm=off  block_type=spram
  Out1 : Outport
  wires:
  Single Port RAM/1 -> Out1/1
  Constant2/1 -> Single Port RAM/3
  In1/1 -> Single Port RAM/2
  Counter/1 -> Single Port RAM/1

== system pfb_fir_real_test/pfb_fir_real/pfb_row_21/delay_bram5 ==
  In1 : Inport
  Constant2 : xbsIndex_r4/Constant  arith_type=Boolean  const=1  n_bits=1  bin_pt=0  explicit_period=on  period=1  equ=P=C  opselect=C  inp2=PCIN>>17  opr=+  inp1=P  carry=CIN  dbl_ovrd=off  block_type=constant
      settings: block_version=11.4
  Counter : xbsIndex_r4/Counter  cnt_type=Count Limited  cnt_to=30  operation=Up  start_count=0  cnt_by_val=1  arith_type=Unsigned  n_bits=5  bin_pt=0  load_pin=off  rst=off  en=off  explicit_period=on  period=1  dbl_ovrd=off  use_behavioral_HDL=off  implementation=DSP48  use_rpm=on  block_type=counter
      settings: block_version=11.4
  Single Port RAM : xbsIndex_r4/Single Port RAM  depth=32  initVector=0  distributed_mem=Block RAM  write_mode=Read Before Write  rst=off  init_reg=0  en=off  latency=1  dbl_ovrd=off  optimize=Area  use_rpm=off  block_type=spram
  Out1 : Outport
  wires:
  Single Port RAM/1 -> Out1/1
  Constant2/1 -> Single Port RAM/3
  In1/1 -> Single Port RAM/2
  Counter/1 -> Single Port RAM/1

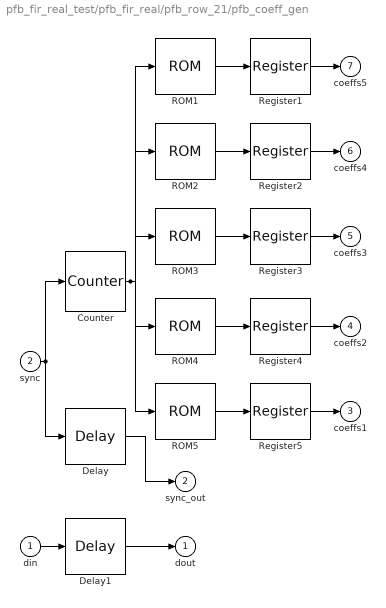
== system pfb_fir_real_test/pfb_fir_real/pfb_row_21/pfb_coeff_gen ==
  din : Inport
  sync : Inport  Port=2
  Counter : xbsIndex_r4/Counter  cnt_type=Free Running  cnt_to=Inf  operation=Up  start_count=0  cnt_by_val=1  arith_type=Unsigned  n_bits=5  bin_pt=0  load_pin=off  rst=on  en=off  explicit_period=on  period=1  dbl_ovrd=off  use_behavioral_HDL=off  implementation=Fabric  use_rpm=on  block_type=counter
      settings: block_version=11.4
  Delay : xbsIndex_r4/Delay  en=off  latency=2  dbl_ovrd=off  reg_retiming=off  block_type=delay
      settings: block_version=11.4
  Delay1 : xbsIndex_r4/Delay  en=off  latency=3  dbl_ovrd=off  reg_retiming=off  block_type=delay
      settings: block_version=11.4
  ROM1 : xbsIndex_r4/ROM  depth=32  initVector=[-1.83537948689192e-20 -5.5570212494937e-06 -1.63600419269467e-05 -3.47242296265235e-05 -6.35238166447315e-05 -0.000106241976471681 -0.000167008217876277 -0.000250618800937326 -0.000362535388329735 -0.000508856971932249 -0.000696260082747423 -0.000931902422689507 -0.00122328536860849 -0.00157807130674446 -0.00200385246963349 -0.002507868871658 -0.00309667407189773 -0.00377574882462827 -0.00454906419223727 -0.00541859736832988 -0.00638380525859058 -0.00744106275440964 -0.00858307456340268 -0.00979827137977639 -0.011070203029117 -0.0123769429460894 -0.0136905198771712 -0.0149763939810333 -0.0161929954652235 -0.017291344491685 -0.0182147712532231 -0.0188987548237974]  distributed_mem=Block RAM  rst=off  init_reg=0  en=off  latency=2  arith_type="Signed  (2's comp)"  n_bits=10  bin_pt=9  dbl_ovrd=off  optimize=Area  use_rpm=on  block_type=sprom
      settings: block_version=11.4
  ROM2 : xbsIndex_r4/ROM  depth=32  initVector=[-0.0192708985824556 -0.0192510586801436 -0.0187516401496287 -0.0176780728545899 -0.0159294765527955 -0.013399520943983 -0.00997748273503472 -0.00554949754803241 9.58776090258162e-18 0.00678665941101795 0.0149244367666534 0.024523677457147 0.0356890847292955 0.0485176039711326 0.0630962566317489 0.0794999611480237 0.0977893811012691 0.118008842950763 0.140184366995717 0.164321855626379 0.190405482381545 0.21839632379788 0.248231273503403 0.279822274484999 0.313055900984824 0.34779331611502 0.383870625110952 0.421099637279897 0.459269042275782 0.498145998490477 0.537478123262804 0.576995866443847]  distributed_mem=Block RAM  rst=off  init_reg=0  en=off  latency=2  arith_type="Signed  (2's comp)"  n_bits=10  bin_pt=9  dbl_ovrd=off  optimize=Area  use_rpm=on  block_type=sprom
      settings: block_version=11.4
  ROM3 : xbsIndex_r4/ROM  depth=32  initVector=[0.616415240804449 0.655440875013837 0.693769347641133 0.731092754011235 0.767102451949175 0.80149292762253 0.83396571896988 0.864233331691149 0.892023081552472 0.917080796874454 0.939174316547831 0.958096721742031 0.973669243595624 0.98574379452744 0.99420507727783 0.998972233248538 1 0.997279356709406 0.990837645797992 0.980738168597035 0.967079262627824 0.949992877609162 0.929642676468857 0.906221696224427 0.879949611428438 0.851069649779872 0.819845215341666 0.786556279459168 0.751495602856677 0.714964854442019 0.67727069304653 0.638720877676221]  distributed_mem=Block RAM  rst=off  init_reg=0  en=off  latency=2  arith_type="Signed  (2's comp)"  n_bits=10  bin_pt=9  dbl_ovrd=off  optimize=Area  use_rpm=on  block_type=sprom
      settings: block_version=11.4
  ROM4 : xbsIndex_r4/ROM  depth=32  initVector=[0.599620469886999 0.560268188690169 0.520952974039709 0.481950809570252 0.443521848986383 0.40590788350912 0.369330180237019 0.333987713358341 0.300055802042386 0.267685160726547 0.237001359579851 0.208104685332775 0.181070385572542 0.155949273151139 0.132768661658431 0.111533598070868 0.0922283547694533 0.0748181401760309 0.0592509853065098 0.0454597625806334 0.0333642932339546 0.0228735006003976 0.0138875683049731 0.00630006494050392 8.87861210313256e-18 -0.00512622041298097 -0.00919296538822508 -0.0123137013214723 -0.0145994824432491 -0.0161576231160187 -0.0170905605431562 -0.017494911978617]  distributed_mem=Block RAM  rst=off  init_reg=0  en=off  latency=2  arith_type="Signed  (2's comp)"  n_bits=10  bin_pt=9  dbl_ovrd=off  optimize=Area  use_rpm=on  block_type=sprom
      settings: block_version=11.4
  ROM5 : xbsIndex_r4/ROM  depth=32  initVector=[-0.017460726222102 -0.0170709252152087 -0.0164009279898009 -0.0155184461159748 -0.0144834371934731 -0.013348200851566 -0.0121576001774965 -0.0109493904773777 -0.00975463676747319 -0.00859820136776993 -0.00749928338318453 -0.00647199266182947 -0.00552594195933946 -0.00466684245382657 -0.00389708938574173 -0.00321632637849668 -0.00262197886823068 -0.00210974897665909 -0.00167406604597449 -0.00130848887129482 -0.00100605737264354 -0.000759593010482301 -0.000561948639457462 -0.000406209694920779 -0.000285849604064716 -0.000194843103417715 -0.000127741728803638 -7.97161304010817e-05 -4.65700670323589e-05 -2.47309672256418e-05 -1.12218300973319e-05 -5.95375857785367e-06]  distributed_mem=Block RAM  rst=off  init_reg=0  en=off  latency=2  arith_type="Signed  (2's comp)"  n_bits=10  bin_pt=9  dbl_ovrd=off  optimize=Area  use_rpm=on  block_type=sprom
      settings: block_version=11.4
  Register{1..5} (5 alike) : xbsIndex_r4/Register  init=0  rst=off  en=off  dbl_ovrd=off  block_type=register
      settings: block_version=11.4
  dout : Outport
  sync_out : Outport  Port=2
  coeffs1 : Outport  Port=3
  coeffs2 : Outport  Port=4
  coeffs3 : Outport  Port=5
  coeffs4 : Outport  Port=6
  coeffs5 : Outport  Port=7
  wires:
  sync/1 -> Delay/1, Counter/1
  Counter/1 -> ROM1/1, ROM2/1, ROM3/1, ROM4/1, ROM5/1
  Register1/1 -> coeffs5/1
  ROM1/1 -> Register1/1
  Register2/1 -> coeffs4/1
  ROM2/1 -> Register2/1
  Register3/1 -> coeffs3/1
  ROM3/1 -> Register3/1
  Register4/1 -> coeffs2/1
  ROM4/1 -> Register4/1
  Register5/1 -> coeffs1/1
  ROM5/1 -> Register5/1
  Delay1/1 -> dout/1
  din/1 -> Delay1/1
  Delay/1 -> sync_out/1

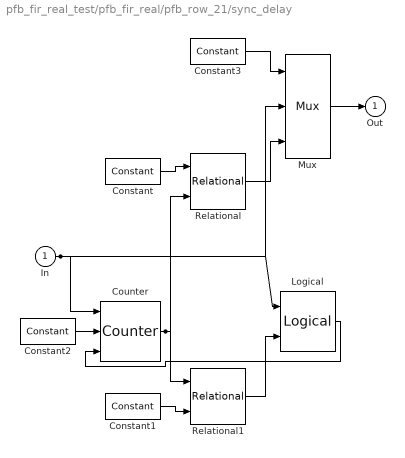
== system pfb_fir_real_test/pfb_fir_real/pfb_row_21/sync_delay ==
  In : Inport
  Constant : xbsIndex_r4/Constant  arith_type=Unsigned  const=1  n_bits=8  bin_pt=0  explicit_period=on  period=1  equ=P=C  opselect=C  inp2=PCIN>>17  opr=+  inp1=P  carry=CIN  dbl_ovrd=off  block_type=constant
      settings: block_version=11.4
  Constant1 : xbsIndex_r4/Constant  arith_type=Unsigned  const=0  n_bits=8  bin_pt=0  explicit_period=on  period=1  equ=P=C  opselect=C  inp2=PCIN>>17  opr=+  inp1=P  carry=CIN  dbl_ovrd=off  block_type=constant
      settings: block_version=11.4
  Constant2 : xbsIndex_r4/Constant  arith_type=Unsigned  const=131  n_bits=8  bin_pt=0  explicit_period=on  period=1  equ=P=C  opselect=C  inp2=PCIN>>17  opr=+  inp1=P  carry=CIN  dbl_ovrd=off  block_type=constant
      settings: block_version=11.4
  Constant3 : xbsIndex_r4/Constant  arith_type=Unsigned  const=1  n_bits=1  bin_pt=0  explicit_period=on  period=1  equ=P=C  opselect=C  inp2=PCIN>>17  opr=+  inp1=P  carry=CIN  dbl_ovrd=off  block_type=constant
      settings: block_version=11.4
  Counter : xbsIndex_r4/Counter  cnt_type=Free Running  cnt_to=Inf  operation=Down  start_count=0  cnt_by_val=1  arith_type=Unsigned  n_bits=8  bin_pt=0  load_pin=on  rst=off  en=on  explicit_period=on  period=1  dbl_ovrd=off  use_behavioral_HDL=off  implementation=Fabric  use_rpm=on  block_type=counter
      settings: block_version=11.4
  Logical : xbsIndex_r4/Logical  logical_function=OR  inputs=2  en=off  latency=0  precision=Full  arith_type=Unsigned  n_bits=16  bin_pt=0  align_bp=on  dbl_ovrd=off  block_type=logical
      settings: block_version=11.4
  Mux : xbsIndex_r4/Mux  inputs=2  en=off  latency=0  precision=Full  arith_type="Signed  (2's comp)"  n_bits=8  bin_pt=2  quantization=Truncate  overflow=Wrap  dbl_ovrd=off  block_type=mux
      settings: block_version=11.4
  Relational : xbsIndex_r4/Relational  mode=a=b  en=off  latency=0  dbl_ovrd=off  block_type=relational
  Relational1 : xbsIndex_r4/Relational  mode=a!=b  en=off  latency=0  dbl_ovrd=off  block_type=relational
  Out : Outport
  wires:
  In/1 -> Mux/2, Logical/1, Counter/1
  Counter/1 -> Relational1/1, Relational/2
  Relational1/1 -> Logical/2
  Constant1/1 -> Relational1/2
  Relational/1 -> Mux/3
  Constant/1 -> Relational/1
  Mux/1 -> Out/1
  Constant3/1 -> Mux/1
  Logical/1 -> Counter/3
  Constant2/1 -> Counter/2

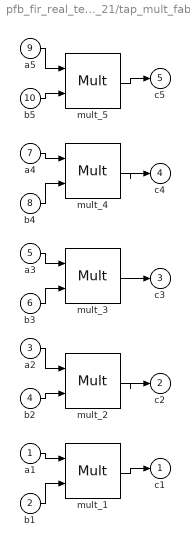
== system pfb_fir_real_test/pfb_fir_real/pfb_row_21/tap_mult_fabric ==
  a1 : Inport
  b1 : Inport  Port=2
  a2 : Inport  Port=3
  b2 : Inport  Port=4
  a3 : Inport  Port=5
  b3 : Inport  Port=6
  a4 : Inport  Port=7
  b4 : Inport  Port=8
  a5 : Inport  Port=9
  b5 : Inport  Port=10
  mult_{1..5} (5 alike) : xbsIndex_r4/Mult  precision=Full  arith_type="Signed  (2's comp)"  n_bits=16  bin_pt=14  quantization=Truncate  overflow=Wrap  en=off  latency=3  dbl_ovrd=off  use_behavioral_HDL=off  opt=Speed  use_embedded=on  optimum_pipeline=off  pipeline=on  use_rpm=on  placement_style=Triangular  block_type=mult
      settings: block_version=11.4
  c1 : Outport
  c2 : Outport  Port=2
  c3 : Outport  Port=3
  c4 : Outport  Port=4
  c5 : Outport  Port=5
  wires:
  mult_5/1 -> c5/1
  b5/1 -> mult_5/2
  a5/1 -> mult_5/1
  mult_4/1 -> c4/1
  b4/1 -> mult_4/2
  a4/1 -> mult_4/1
  mult_3/1 -> c3/1
  b3/1 -> mult_3/2
  a3/1 -> mult_3/1
  mult_2/1 -> c2/1
  b2/1 -> mult_2/2
  a2/1 -> mult_2/1
  mult_1/1 -> c1/1
  b1/1 -> mult_1/2
  a1/1 -> mult_1/1
